simulink model "friction_model"  (R2023a)
settings: Solver=VariableStepAuto  StartTime=0.0  StopTime=10.0  RelTol=1e-3
values from neighbouring files (symbols this model uses):
  b = 15.2092    [modelsetup.m]
  currents = data(:, 2)    [modelevaluation.m]    (also in modelsetup.m)
  dt = mean(diffs)    [modelevaluation.m]    (also in modelsetup.m)
  EPSILON = 0.005    [modelsetup.m]
  F_c = 13.4362    [modelsetup.m]
  F_stat = 11.9040    (= 11.904)    [modelsetup.m]
  J = 5.0652    [modelsetup.m]
  K_t = 14.88    [modelsetup.m]
settings Model: Creator=yunzh  LastModifiedBy=yunzh

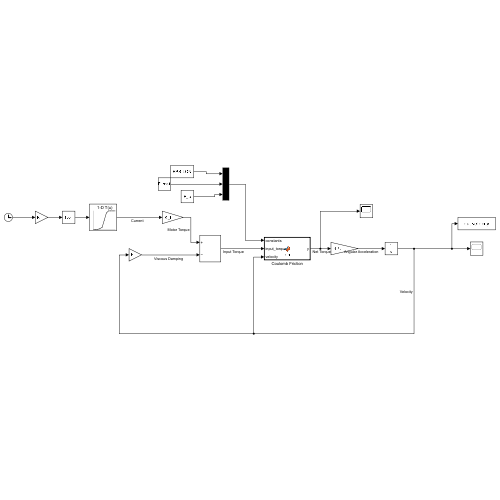
[thumbnail: Simulink's stored preview of the top-level diagram]
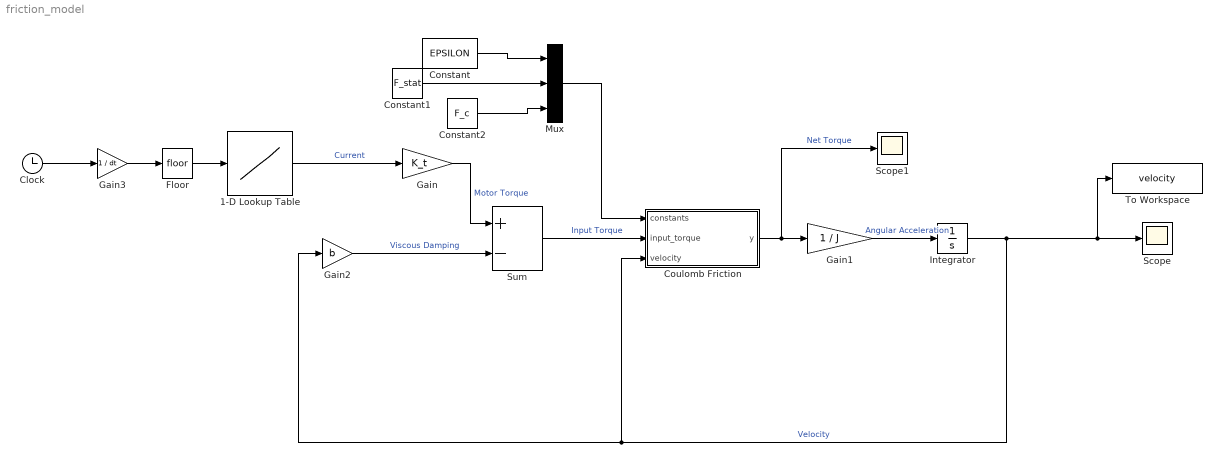
== system friction_model ==
  1-D Lookup Table : Lookup_n-D  NumberOfTableDimensions=1  BreakpointsForDimension1=[1:numel(currents)]'  Table=currents  InternalRulePriority=Speed  RndMeth=Simplest
  Clock : Clock
  Constant : Constant  Value=EPSILON
  Constant1 : Constant  Value=F_stat
  Constant2 : Constant  Value=F_c
  Coulomb Friction : MATLAB Function  TreatAsAtomicUnit=on
  Floor : Rounding
  Gain : Gain  Gain=K_t
  Gain1 : Gain  Gain=1 / J
  Gain2 : Gain  Gain=b
  Gain3 : Gain  Gain=1 / dt
  Integrator : Integrator
  Mux : Mux  Inputs=3
  Scope : Scope
  Scope1 : Scope
  Sum : Sum  Inputs=+-
  To Workspace : ToWorkspace  VariableName=velocity  SaveFormat=Timeseries  SampleTime=-1
  wires:
  Gain/1 -> Sum/1  "Motor Torque"
  1-D Lookup Table/1 -> Gain/1  "Current"
  Gain2/1 -> Sum/2  "Viscous Damping"
  Gain1/1 -> Integrator/1  "Angular Acceleration"
  Integrator/1 -> Gain2/1, Coulomb Friction/3(velocity), To Workspace/1, Scope/1  "Velocity"
  Sum/1 -> Coulomb Friction/2(input_torque)  "Input Torque"
  Coulomb Friction/1(y) -> Scope1/1, Gain1/1  "Net Torque"
  Mux/1 -> Coulomb Friction/1(constants)
  Constant/1 -> Mux/1
  Constant2/1 -> Mux/3
  Constant1/1 -> Mux/2
  Floor/1 -> 1-D Lookup Table/1
  Gain3/1 -> Floor/1
  Clock/1 -> Gain3/1

== matlab function friction_model/Coulomb Friction ==
  data: constants input; input_torque input; velocity input; y output
function y = fcn(constants, input_torque, velocity)
    EPSILON = constants(1);
    F_stat = constants(2);
    F_c = constants(3);


    if abs(velocity) < EPSILON % no motion
        if abs(input_torque) < abs(F_stat) % insufficient torque
            y = 0;
            return
        end

        % reduce torque by static friction
        static_friction = -1 * sign(input_torque) * F_stat;
        y = input_torque + static_friction;
        return
    end
    
    % reduce torque by dynamic friction
    dynamic_friction = -1 * sign(velocity) * F_c;
    y = input_torque + dynamic_friction;
end
